simulink subsystem "DirectDriveCycle_refsub"  (R2022a)
settings: Solver=VariableStepAuto  StartTime=0.0  StopTime=10.0  RelTol=1e-3
undefined symbols (not defined in the file or in its folder): bevControl, motorDrive, vehicle
libraries: autolibshared x1
settings Model: Creator=isaacito  LastModifiedBy=isaacito
settings SolverCC: AlgebraicLoopSolver=TrustRegion
settings DebuggingCC: UnconnectedInputMsg=warning  UnconnectedOutputMsg=warning  UnconnectedLineMsg=warning  SFMachineParentedDataDiag=warning
settings RTWCC: DLArmComputeVersion=19.05

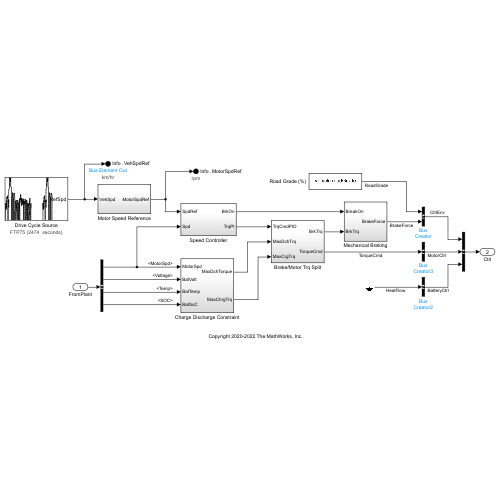
[thumbnail: Simulink's stored preview of the top-level diagram]
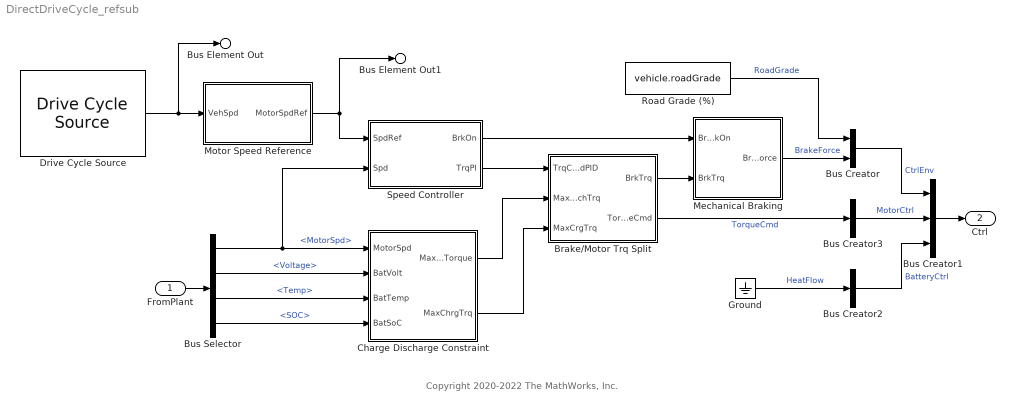
== system DirectDriveCycle_refsub ==
  note: Copyright 2020-2022 The MathWorks, Inc.
  FromPlant : Inport
  Brake/Motor Trq Split : Subsystem
  Bus Creator : BusCreator  Inputs=2
  Bus Creator1 : BusCreator  Inputs=3
  Bus Creator2 : BusCreator  Inputs=1
  Bus Creator3 : BusCreator  Inputs=1
  Bus Selector : BusSelector  OutputSignals=Motor.MotorSpd,Battery.Voltage,Battery.Temp,Battery.SOC
  Charge Discharge Constraint : Subsystem
  Drive Cycle Source : autolibshared/Drive Cycle Source  cycleVar=FTP75  fileVar=cycleFTP75.mat  tfinal="2474  seconds"  cycleRepeat=off  outAccPort=off  outGearPort=off  gearList=No gear data  t_wot1=5  xdot_woto=0  xdot_wot1=30  t_wot2=20  xdot_wot2=0  t_wotend=30  srcUnit=m/s  outUnit=km/h  srcAccUnit=m/s/s  outAccUnit=m/s^2  dt=0  aMode=1  faultOption=off  velBnd=2  velBndUnit=mph  inUnit=m/s  timeBnd=1  failOption=off  stopSim=off  maxFaultCnt=10  maxFaultTime=2  maxTotFaultTime=15  traceOption=off  dtTrace=1  traceWindow=10  lastDCname=FTP75  lastOutUnit=mph  lastDT=0  lastTB=1  lastSB=2  forceCalcBound=off
      settings: SourceProductBaseCode=PW,DR,MT,VE
  Ground : Ground
  Mechanical Braking : Subsystem
  Motor Speed Reference : Subsystem
  Road Grade (%) : Constant  Value=vehicle.roadGrade
  Speed Controller : Subsystem
      settings: PortSchema="{\"entries\":[{\"content\":{\"sides\":[{\"content\":{\"connectorIds\":[\"Out1\",\"Out2\"]},\"type\":\"ConnectorPlacement.EquallySpacedRectSide\",\"uuid\":\"12b9f2c9-2b28-451b-ad36-7fe4150db485\"},{\"content\":{\"connectorIds\":[\"In1\",\"In2\"],\"side\":\"RIGHT\"},\"type\":\"ConnectorPlacement.EquallySpacedRectSide\",\"uuid\":\"c0fdf9a4-483a-4ddc-b663-6299fcc79327\"},{\"content\":{\"connectorIds\":[],\"side\":\"TOP\"},\"type\":\"ConnectorPlacement.EquallySpacedRectSide\",\"uuid\":\"3f20082e-8487-45e3-9fd7-d6d75741df4d\"}]},\"type\":\"ConnectorPlacement.EquallySpacedConnector\",\"uuid\":\"9361cdd3-74d8-46ee-ae7f-e2dde5d31ed1\"}],\"packageUris\":[\"http://schema.mathworks.com/mf0/Connector/R2020b\"],\"version\":\"1.0\"}"
  Bus Element Out : Outport  PortName=Info  Element=VehSpdRef
      settings: AttributesFormatString=%<Unit>
  Bus Element Out1 : Outport  PortName=Info  Element=MotorSpdRef
      settings: AttributesFormatString=%<Unit>
  Ctrl : Outport  Port=2
  wires:
  Drive Cycle Source/1 -> Bus Element Out/1, Motor Speed Reference/1(VehSpd)
  FromPlant/1 -> Bus Selector/1
  Bus Selector/1 -> Charge Discharge Constraint/1(MotorSpd), Speed Controller/2(Spd)  "<MotorSpd>"
  Ground/1 -> Bus Creator2/1  "HeatFlow"
  Bus Creator/1 -> Bus Creator1/1  "CtrlEnv"
  Bus Creator3/1 -> Bus Creator1/2  "MotorCtrl"
  Bus Creator2/1 -> Bus Creator1/3  "BatteryCtrl"
  Bus Creator1/1 -> Ctrl/1
  Speed Controller/2(TrqPI) -> Brake/Motor Trq Split/1(TrqCmdPID)
  Speed Controller/1(BrkOn) -> Mechanical Braking/1(BreakOn)
  Charge Discharge Constraint/1(MaxDchTorque) -> Brake/Motor Trq Split/2(MaxDchTrq)
  Charge Discharge Constraint/2(MaxChrgTrq) -> Brake/Motor Trq Split/3(MaxCrgTrq)
  Brake/Motor Trq Split/1(BrkTrq) -> Mechanical Braking/2(BrkTrq)
  Brake/Motor Trq Split/2(TorqueCmd) -> Bus Creator3/1  "TorqueCmd"
  Bus Selector/3 -> Charge Discharge Constraint/3(BatTemp)  "<Temp>"
  Bus Selector/4 -> Charge Discharge Constraint/4(BatSoC)  "<SOC>"
  Motor Speed Reference/1(MotorSpdRef) -> Bus Element Out1/1, Speed Controller/1(SpdRef)
  Bus Selector/2 -> Charge Discharge Constraint/2(BatVolt)  "<Voltage>"
  Mechanical Braking/1(BrakeForce) -> Bus Creator/2  "BrakeForce"
  Road Grade (%)/1 -> Bus Creator/1  "RoadGrade"

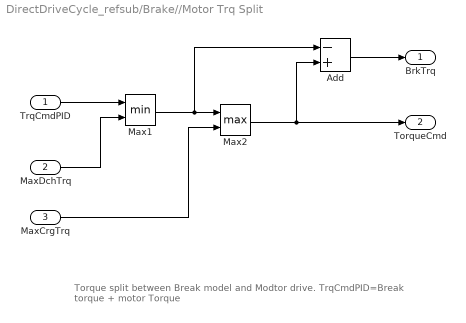
== system DirectDriveCycle_refsub/Brake//Motor Trq Split ==
  note: Torque split between Break model and Modtor drive.
      | TrqCmdPID=Break torque + motor Torque
  TrqCmdPID : Inport
  MaxDchTrq : Inport  Port=2
  MaxCrgTrq : Inport  Port=3
  Add : Sum  Inputs=-+
  Max1 : MinMax  Inputs=2  ZeroCross=off
  Max2 : MinMax  Function=max  Inputs=2  ZeroCross=off
  BrkTrq : Outport
  TorqueCmd : Outport  Port=2
  wires:
  MaxDchTrq/1 -> Max1/2
  Max2/1 -> Add/2, TorqueCmd/1
  Add/1 -> BrkTrq/1
  Max1/1 -> Add/1, Max2/1
  TrqCmdPID/1 -> Max1/1
  MaxCrgTrq/1 -> Max2/2

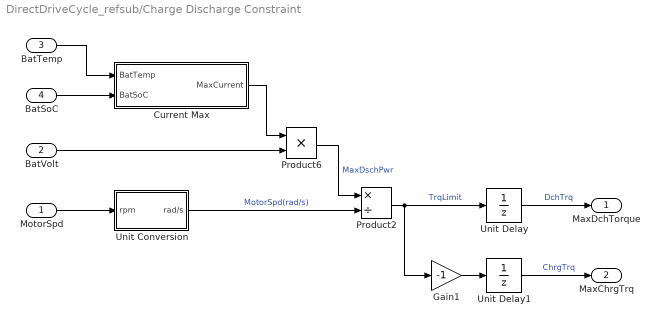
== system DirectDriveCycle_refsub/Charge Discharge Constraint ==
  MotorSpd : Inport
  BatVolt : Inport  Port=2
  BatTemp : Inport  Port=3
  BatSoC : Inport  Port=4
  Current Max : Subsystem
  Gain1 : Gain  Gain=-1
  Product2 : Product  Inputs=*/
  Product6 : Product
  Unit Conversion : Subsystem
  Unit Delay : UnitDelay  InitialCondition=eps  SampleTime=-1  HasFrameUpgradeWarning=on
  Unit Delay1 : UnitDelay  InitialCondition=eps  SampleTime=-1  HasFrameUpgradeWarning=on
  MaxDchTorque : Outport
  MaxChrgTrq : Outport  Port=2
  wires:
  Gain1/1 -> Unit Delay1/1
  Current Max/1(MaxCurrent) -> Product6/1
  BatSoC/1 -> Current Max/2(BatSoC)
  BatTemp/1 -> Current Max/1(BatTemp)
  MotorSpd/1 -> Unit Conversion/1(rpm)
  Unit Conversion/1(rad/s) -> Product2/2  "MotorSpd(rad/s)"
  Product6/1 -> Product2/1  "MaxDschPwr"
  Product2/1 -> Unit Delay/1, Gain1/1  "TrqLimit"
  BatVolt/1 -> Product6/2
  Unit Delay1/1 -> MaxChrgTrq/1  "ChrgTrq"
  Unit Delay/1 -> MaxDchTorque/1  "DchTrq"

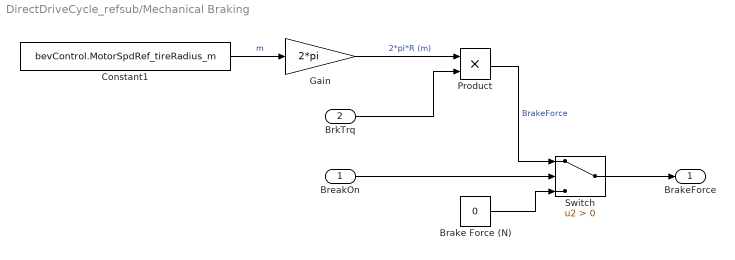
== system DirectDriveCycle_refsub/Mechanical Braking ==
  BreakOn : Inport
  BrkTrq : Inport  Port=2
  Brake Force (N) : Constant  Value=0
  Constant1 : Constant  Value=bevControl.MotorSpdRef_tireRadius_m
  Gain : Gain  Gain=2*pi
  Product : Product
  Switch : Switch  Criteria=u2 > Threshold  ZeroCross=off  SaturateOnIntegerOverflow=off  InputSameDT=off
  BrakeForce : Outport
  wires:
  Switch/1 -> BrakeForce/1
  Constant1/1 -> Gain/1  "m"
  Brake Force (N)/1 -> Switch/3
  BreakOn/1 -> Switch/2
  BrkTrq/1 -> Product/2
  Gain/1 -> Product/1  "2*pi*R (m)"
  Product/1 -> Switch/1  "BrakeForce"

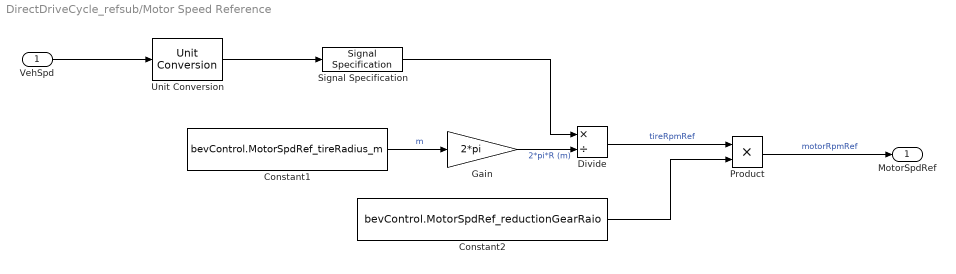
== system DirectDriveCycle_refsub/Motor Speed Reference ==
  VehSpd : Inport  Unit=km/hr
  Constant1 : Constant  Value=bevControl.MotorSpdRef_tireRadius_m
  Constant2 : Constant  Value=bevControl.MotorSpdRef_reductionGearRaio
  Divide : Product  Inputs=*/
  Gain : Gain  Gain=2*pi
  Product : Product
  Signal Specification : SignalSpecification  Unit=m/min
  Unit Conversion : UnitConversion
  MotorSpdRef : Outport  Unit=rpm  VectorParamsAs1DForOutWhenUnconnected=off
  wires:
  Constant1/1 -> Gain/1  "m"
  Product/1 -> MotorSpdRef/1  "motorRpmRef"
  Constant2/1 -> Product/2
  Divide/1 -> Product/1  "tireRpmRef"
  Gain/1 -> Divide/2  "2*pi*R (m)"
  Signal Specification/1 -> Divide/1
  Unit Conversion/1 -> Signal Specification/1
  VehSpd/1 -> Unit Conversion/1

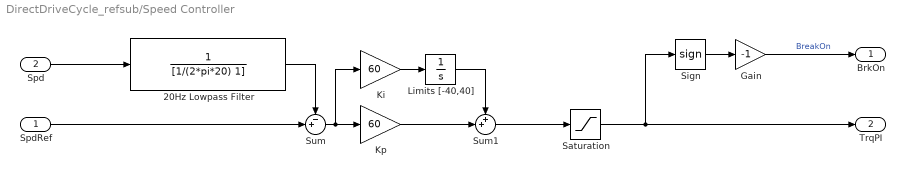
== system DirectDriveCycle_refsub/Speed Controller ==
  SpdRef : Inport  Unit=rpm
      settings: AttributesFormatString=%<Unit>
  Spd : Inport  Port=2  Unit=rpm
      settings: AttributesFormatString=%<Unit>
  20Hz Lowpass Filter : TransferFcn  Denominator=[1/(2*pi*20) 1]
  Gain : Gain  Gain=-1
  Ki : Gain  Gain=60
  Kp : Gain  Gain=60
  Limits [-40,40] : Integrator  LimitOutput=on  UpperSaturationLimit=40  LowerSaturationLimit=-40
  Saturation : Saturate  UpperLimit=motorDrive.simplePmsmDrv_trqMax_Nm  LowerLimit=-motorDrive.simplePmsmDrv_trqMax_Nm
      settings: AttributesFormatString=|
      | %<UpperLimit>
      | %<LowerLimit>
  Sign : Signum  ZeroCross=off
  Sum : Sum  Inputs=-+|
  Sum1 : Sum  Inputs=++|
  BrkOn : Outport
  TrqPI : Outport  Port=2  Unit=N*m  VectorParamsAs1DForOutWhenUnconnected=off
      settings: AttributesFormatString=%<Unit>
  wires:
  Sign/1 -> Gain/1
  Saturation/1 -> TrqPI/1, Sign/1
  Gain/1 -> BrkOn/1  "BreakOn"
  SpdRef/1 -> Sum/2
  Spd/1 -> 20Hz Lowpass Filter/1
  Sum1/1 -> Saturation/1
  Sum/1 -> Ki/1, Kp/1
  Ki/1 -> Limits [-40,40]/1
  Kp/1 -> Sum1/2
  Limits [-40,40]/1 -> Sum1/1
  20Hz Lowpass Filter/1 -> Sum/1

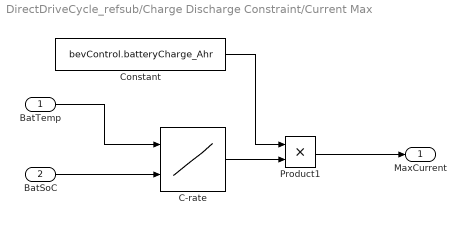
== system DirectDriveCycle_refsub/Charge Discharge Constraint/Current Max ==
  BatTemp : Inport
  BatSoC : Inport  Port=2
  C-rate : Lookup_n-D  BreakpointsForDimension1=bevControl.batteryTemp_LUT  BreakpointsForDimension2=bevControl.batterySOC_LUT  Table=bevControl.cRate'  ExtrapMethod=Clip  UseLastTableValue=on  InternalRulePriority=Speed  RndMeth=Simplest
      settings: InputPortMap=u0,u1
  Constant : Constant  Value=bevControl.batteryCharge_Ahr
  Product1 : Product
  MaxCurrent : Outport
  wires:
  Constant/1 -> Product1/1
  BatSoC/1 -> C-rate/2
  BatTemp/1 -> C-rate/1
  Product1/1 -> MaxCurrent/1
  C-rate/1 -> Product1/2

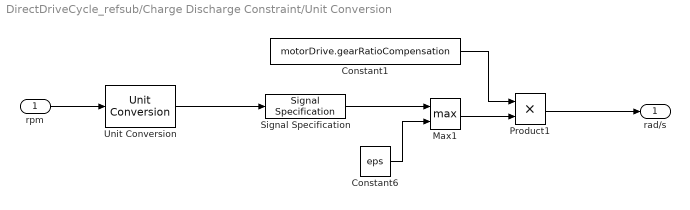
== system DirectDriveCycle_refsub/Charge Discharge Constraint/Unit Conversion ==
  rpm : Inport
  Constant1 : Constant  Value=motorDrive.gearRatioCompensation
  Constant6 : Constant  Value=eps
  Max1 : MinMax  Function=max  Inputs=2  ZeroCross=off
  Product1 : Product
  Signal Specification : SignalSpecification  OutMin=[0]  Unit=rad/sec
  Unit Conversion : UnitConversion
  rad/s : Outport
  wires:
  rpm/1 -> Unit Conversion/1
  Constant1/1 -> Product1/1
  Unit Conversion/1 -> Signal Specification/1
  Max1/1 -> Product1/2
  Product1/1 -> rad/s/1
  Constant6/1 -> Max1/2
  Signal Specification/1 -> Max1/1
